simulink model "Modelo_MV_CIGRE_IPSD"  (R2019b)
settings: Solver=FixedStepAuto  StartTime=0.0  StopTime=0.3  FixedStep=Ts  RelTol=1e-3
PreLoadFcn:
  | r_1=0.501
  | l_1=0.716/(60*2*pi)
  | c_1=10e-6/(60*2*pi)
  | r_0=0.817
  | l_0=1.598 /(60*2*pi)
  | c_0=10e-6/(60*2*pi)
  | Sb=50e6
  | Ts=1e-4
InitFcn:
  | r_1=0.501;
  | l_1=0.716/(60*2*pi);
  | c_1=10e-6/(60*2*pi);
  | r_0=0.817;
  | l_0=1.598 /(60*2*pi);
  | c_0=10e-6/(60*2*pi);
  | Sb=50e6;
  | Ts=1e-4;
StartFcn:
  | r_1=0.501
  | l_1=0.716/(60*2*pi)
  | c_1=10e-6/(60*2*pi)
  | r_0=0.817
  | l_0=1.598 /(60*2*pi)
  | c_0=10e-6/(60*2*pi)
  | Sb=50e6
  | Ts=1e-5
undefined symbols (not defined in the file): D1, Delta
libraries: powerlib_meascontrol x112, powerlib x55, simulink x6
(part 1 of 3)
settings Model: Creator=mance  LastModifiedBy=mance

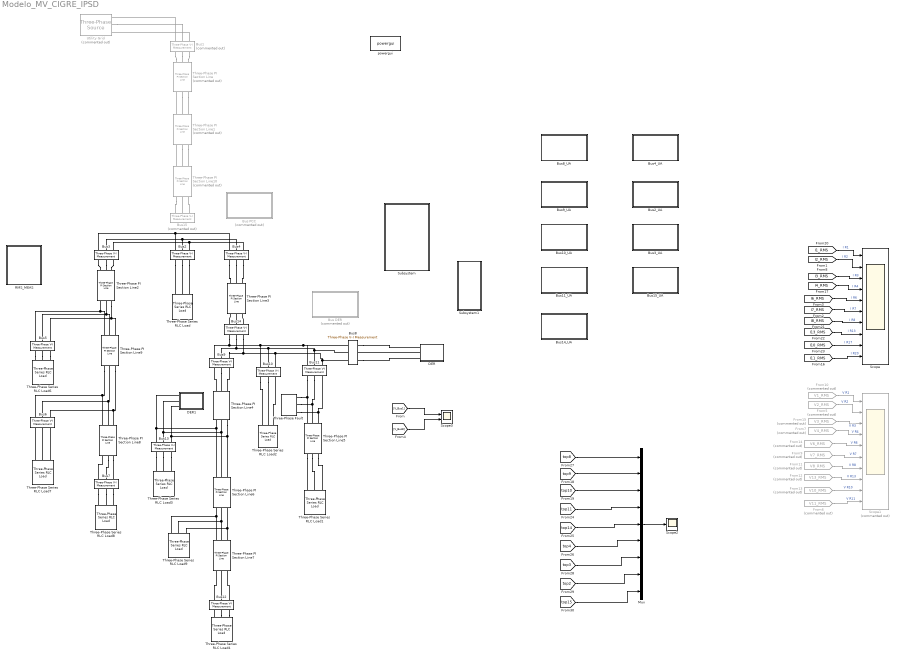
== system Modelo_MV_CIGRE_IPSD ==
  Bus DER : Subsystem  Commented=on
  Bus PCC : Subsystem  Commented=on
  Bus1 : powerlib/Measurements/Three-Phase V-I Measurement  Commented=on  VoltageMeasurement=phase-to-ground  SetLabelV=on  LabelV=V_Bus1  Vpu=on  VpuLL=off  CurrentMeasurement=yes  SetLabelI=on  LabelI=I_Bus1  Ipu=on  Pbase=Sb  Vbase=20e3  OutputType=Complex  PhasorSimulation=off  PSBequivalent=0
      settings: SourceProductName=Simscape Electrical
  Bus10 : powerlib/Measurements/Three-Phase V-I Measurement  VoltageMeasurement=phase-to-ground  SetLabelV=on  LabelV=V_Bus10  Vpu=on  VpuLL=off  CurrentMeasurement=yes  SetLabelI=on  LabelI=I_Bus10  Ipu=on  Pbase=Sb  Vbase=20e3  OutputType=Complex  PhasorSimulation=off  PSBequivalent=0
      settings: SourceProductName=Simscape Electrical
  Bus10_UA : Subsystem
  Bus11 : powerlib/Measurements/Three-Phase V-I Measurement  VoltageMeasurement=phase-to-ground  SetLabelV=on  LabelV=V_Bus11  Vpu=on  VpuLL=off  CurrentMeasurement=yes  SetLabelI=on  LabelI=I_Bus11  Ipu=on  Pbase=Sb  Vbase=20e3  OutputType=Complex  PhasorSimulation=off  PSBequivalent=0
      settings: SourceProductName=Simscape Electrical
  Bus11_UA : Subsystem
  Bus12 : powerlib/Measurements/Three-Phase V-I Measurement  VoltageMeasurement=phase-to-ground  SetLabelV=on  LabelV=V_Bus12  Vpu=on  VpuLL=off  CurrentMeasurement=yes  SetLabelI=on  LabelI=I_Bus12  Ipu=on  Pbase=Sb  Vbase=20e3  OutputType=Complex  PhasorSimulation=off  PSBequivalent=0
      settings: SourceProductName=Simscape Electrical
  Bus13 : powerlib/Measurements/Three-Phase V-I Measurement  VoltageMeasurement=phase-to-ground  SetLabelV=on  LabelV=V_Bus13  Vpu=on  VpuLL=off  CurrentMeasurement=yes  SetLabelI=on  LabelI=I_Bus13  Ipu=on  Pbase=Sb  Vbase=20e3  OutputType=Complex  PhasorSimulation=off  PSBequivalent=0
      settings: SourceProductName=Simscape Electrical
  Bus14 : powerlib/Measurements/Three-Phase V-I Measurement  VoltageMeasurement=phase-to-ground  SetLabelV=on  LabelV=V_Bus14  Vpu=on  VpuLL=off  CurrentMeasurement=yes  SetLabelI=on  LabelI=I_Bus14  Ipu=on  Pbase=Sb  Vbase=20e3  OutputType=Complex  PhasorSimulation=off  PSBequivalent=0
      settings: SourceProductName=Simscape Electrical
  Bus14_UA : Subsystem
  Bus15 : powerlib/Measurements/Three-Phase V-I Measurement  Commented=on  VoltageMeasurement=phase-to-ground  SetLabelV=on  LabelV=V_Bus15  Vpu=on  VpuLL=off  CurrentMeasurement=yes  SetLabelI=on  LabelI=I_Bus15  Ipu=on  Pbase=Sb  Vbase=20e3  OutputType=Complex  PhasorSimulation=off  PSBequivalent=0
      settings: SourceProductName=Simscape Electrical
  Bus15_UA : Subsystem
  Bus2 : powerlib/Measurements/Three-Phase V-I Measurement  VoltageMeasurement=phase-to-ground  SetLabelV=on  LabelV=V_Bus2  Vpu=on  VpuLL=off  CurrentMeasurement=yes  SetLabelI=on  LabelI=I_Bus2  Ipu=on  Pbase=Sb  Vbase=20e3  OutputType=Complex  PhasorSimulation=off  PSBequivalent=0
      settings: SourceProductName=Simscape Electrical
  Bus2_UA : Subsystem
  Bus3 : powerlib/Measurements/Three-Phase V-I Measurement  VoltageMeasurement=phase-to-ground  SetLabelV=on  LabelV=V_Bus3  Vpu=on  VpuLL=off  CurrentMeasurement=yes  SetLabelI=on  LabelI=I_Bus3  Ipu=on  Pbase=Sb  Vbase=20e3  OutputType=Complex  PhasorSimulation=off  PSBequivalent=0
      settings: SourceProductName=Simscape Electrical
  Bus3_UA : Subsystem
  Bus4 : powerlib/Measurements/Three-Phase V-I Measurement  VoltageMeasurement=phase-to-ground  SetLabelV=on  LabelV=V_Bus4  Vpu=on  VpuLL=off  CurrentMeasurement=yes  SetLabelI=on  LabelI=I_Bus4  Ipu=on  Pbase=Sb  Vbase=20e3  OutputType=Complex  PhasorSimulation=off  PSBequivalent=0
      settings: SourceProductName=Simscape Electrical
  Bus4_UA : Subsystem
  Bus5 : powerlib/Measurements/Three-Phase V-I Measurement  VoltageMeasurement=phase-to-ground  SetLabelV=on  LabelV=V_Bus5  Vpu=on  VpuLL=off  CurrentMeasurement=yes  SetLabelI=on  LabelI=I_Bus5  Ipu=on  Pbase=Sb  Vbase=20e3  OutputType=Complex  PhasorSimulation=off  PSBequivalent=0
      settings: SourceProductName=Simscape Electrical
  Bus6 : powerlib/Measurements/Three-Phase V-I Measurement  VoltageMeasurement=phase-to-ground  SetLabelV=on  LabelV=V_Bus6  Vpu=on  VpuLL=off  CurrentMeasurement=yes  SetLabelI=on  LabelI=I_Bus6  Ipu=on  Pbase=Sb  Vbase=20e3  OutputType=Complex  PhasorSimulation=off  PSBequivalent=0
      settings: SourceProductName=Simscape Electrical
  Bus7 : powerlib/Measurements/Three-Phase V-I Measurement  VoltageMeasurement=phase-to-ground  SetLabelV=on  LabelV=V_Bus7  Vpu=on  VpuLL=off  CurrentMeasurement=yes  SetLabelI=on  LabelI=I_Bus7  Ipu=on  Pbase=Sb  Vbase=20e3  OutputType=Complex  PhasorSimulation=off  PSBequivalent=0
      settings: SourceProductName=Simscape Electrical
  Bus8 : powerlib/Measurements/Three-Phase V-I Measurement  VoltageMeasurement=phase-to-ground  SetLabelV=on  LabelV=V_Bus8  Vpu=on  VpuLL=off  CurrentMeasurement=yes  SetLabelI=on  LabelI=I_Bus8  Ipu=on  Pbase=Sb  Vbase=20e3  OutputType=Complex  PhasorSimulation=off  PSBequivalent=0
      settings: SourceProductName=Simscape Electrical
  Bus8_UA : Subsystem
  Bus9 : powerlib/Measurements/Three-Phase V-I Measurement  VoltageMeasurement=phase-to-ground  SetLabelV=on  LabelV=V_Bus9  Vpu=on  VpuLL=off  CurrentMeasurement=yes  SetLabelI=on  LabelI=I_Bus9  Ipu=on  Pbase=Sb  Vbase=20e3  OutputType=Complex  PhasorSimulation=off  PSBequivalent=0
      settings: SourceProductName=Simscape Electrical
  Bus9_UA : Subsystem
  DER : Subsystem
  DER1 : Subsystem
  From10 : From  Commented=on  GotoTag=V1_RMS  TagVisibility=global
  From11 : From  Commented=on  GotoTag=V8_RMS  TagVisibility=global
  From12 : From  Commented=on  GotoTag=V13_RMS  TagVisibility=global
  From13 : From  Commented=on  GotoTag=V10_RMS  TagVisibility=global
  From14 : From  Commented=on  GotoTag=V6_RMS  TagVisibility=global
  From15 : From  Commented=on  GotoTag=V3_RMS  TagVisibility=global
  From5 : From  Commented=on  GotoTag=V2_RMS  TagVisibility=global
  From6 : From  Commented=on  GotoTag=V11_RMS  TagVisibility=global
  From7 : From  Commented=on  GotoTag=V4_RMS  TagVisibility=global
  From9 : From  Commented=on  GotoTag=V7_RMS  TagVisibility=global
  Mux : Mux  Inputs=9
  RMS_MEAS : Subsystem
  Scope : Scope  NumInputPorts=10
  Scope1 : Scope  Commented=on  NumInputPorts=10
  Scope2 : Scope
  Scope3 : Scope  NumInputPorts=2
  Subsystem : Subsystem
  Subsystem1 : Subsystem
  Three-Phase PI Section Line : powerlib/Elements/Three-Phase PI Section Line  Commented=on  LConnTagsString=a|b|c  RConnTagsString=A|B|C  Frequency=60  Resistances=[ r_1 r_0]  Inductances=[ l_1 l_0]  Capacitances=[c_1 c_0]  Length=1.2
      settings: SourceProductName=Simscape Electrical
  Three-Phase PI Section Line1 : powerlib/Elements/Three-Phase PI Section Line  Commented=on  LConnTagsString=a|b|c  RConnTagsString=A|B|C  Frequency=60  Resistances=[r_1 r_0]  Inductances=[l_1 l_0]  Capacitances=[c_1 c_0]  Length=0.5
      settings: SourceProductName=Simscape Electrical
  Three-Phase PI Section Line10 : powerlib/Elements/Three-Phase PI Section Line  Commented=on  LConnTagsString=a|b|c  RConnTagsString=A|B|C  Frequency=60  Resistances=[r_1 r_0]  Inductances=[l_1 l_0]  Capacitances=[c_1 c_0]  Length=0.5
      settings: SourceProductName=Simscape Electrical
  Three-Phase PI Section Line2 : powerlib/Elements/Three-Phase PI Section Line  LConnTagsString=a|b|c  RConnTagsString=A|B|C  Frequency=60  Resistances=[r_1 r_0]  Inductances=[l_1 l_0]  Capacitances=[c_1 c_0]  Length=0.6
      settings: SourceProductName=Simscape Electrical
  Three-Phase PI Section Line3 : powerlib/Elements/Three-Phase PI Section Line  LConnTagsString=a|b|c  RConnTagsString=A|B|C  Frequency=60  Resistances=[r_1 r_0]  Inductances=[l_1 l_0]  Capacitances=[c_1 c_0]  Length=1.3
      settings: SourceProductName=Simscape Electrical
  Three-Phase PI Section Line4 : powerlib/Elements/Three-Phase PI Section Line  LConnTagsString=a|b|c  RConnTagsString=A|B|C  Frequency=60  Resistances=[r_1 r_0]  Inductances=[l_1 l_0]  Capacitances=[c_1 c_0]  Length=0.3
      settings: SourceProductName=Simscape Electrical
  Three-Phase PI Section Line5 : powerlib/Elements/Three-Phase PI Section Line  LConnTagsString=a|b|c  RConnTagsString=A|B|C  Frequency=60  Resistances=[r_1 r_0]  Inductances=[l_1 l_0]  Capacitances=[c_1 c_0]  Length=1.7
      settings: SourceProductName=Simscape Electrical
  Three-Phase PI Section Line6 : powerlib/Elements/Three-Phase PI Section Line  LConnTagsString=a|b|c  RConnTagsString=A|B|C  Frequency=60  Resistances=[r_1 r_0]  Inductances=[l_1 l_0]  Capacitances=[c_1 c_0]  Length=0.8
      settings: SourceProductName=Simscape Electrical
  Three-Phase PI Section Line7 : powerlib/Elements/Three-Phase PI Section Line  LConnTagsString=a|b|c  RConnTagsString=A|B|C  Frequency=60  Resistances=[r_1 r_0]  Inductances=[l_1 l_0]  Capacitances=[c_1 c_0]  Length=0.3
      settings: SourceProductName=Simscape Electrical
  Three-Phase PI Section Line8 : powerlib/Elements/Three-Phase PI Section Line  LConnTagsString=a|b|c  RConnTagsString=A|B|C  Frequency=60  Resistances=[r_1 r_0]  Inductances=[l_1 l_0]  Capacitances=[c_1 c_0]  Length=1.5
      settings: SourceProductName=Simscape Electrical
  Three-Phase PI Section Line9 : powerlib/Elements/Three-Phase PI Section Line  LConnTagsString=a|b|c  RConnTagsString=A|B|C  Frequency=60  Resistances=[r_1 r_0]  Inductances=[l_1 l_0]  Capacitances=[c_1 c_0]  Length=0.6
      settings: SourceProductName=Simscape Electrical
  Three-Phase Series RLC Load : powerlib/Elements/Three-Phase Series RLC Load  LConnTagsString=A|B|C  Configuration=Y (grounded)  NominalVoltage=(20000)  Vabc=[1e3 1e3 1e3]  Vabcp=[1e3 1e3 1e3]  NominalFrequency=60  UnbalancedPower=off  ActivePower=15e3*0.9  InductivePower=sqrt(15e3^2-(15e3*0.9)^2)  CapacitivePower=0  Pabc=[10e3 9e3 11e3]  QLabc=[100 90 110]  QCabc=[100 90 110]  Pabcp=[10e3 9e3 11e3]  QLabcp=[100 90 110]  QCabcp=[100 90 110]  Measurements=None  LoadType=constant PQ
      settings: SourceProductName=Simscape Electrical
  Three-Phase Series RLC Load1 : powerlib/Elements/Three-Phase Series RLC Load  LConnTagsString=A|B|C  Configuration=Y (grounded)  NominalVoltage=(20000)  Vabc=[1e3 1e3 1e3]  Vabcp=[1e3 1e3 1e3]  NominalFrequency=60  UnbalancedPower=off  ActivePower=50e3*0.95*0.7  InductivePower=sqrt(50e3^2-(50e3*0.95)^2)*0.7  CapacitivePower=0  Pabc=[10e3 9e3 11e3]  QLabc=[100 90 110]  QCabc=[100 90 110]  Pabcp=[10e3 9e3 11e3]  QLabcp=[100 90 110]  QCabcp=[100 90 110]  Measurements=None  LoadType=constant PQ
      settings: SourceProductName=Simscape Electrical
  Three-Phase Series RLC Load2 : powerlib/Elements/Three-Phase Series RLC Load  LConnTagsString=A|B|C  Configuration=Y (grounded)  NominalVoltage=(20000)  Vabc=[1e3 1e3 1e3]  Vabcp=[1e3 1e3 1e3]  NominalFrequency=60  UnbalancedPower=off  ActivePower=10e3*0.95*0.7  InductivePower=sqrt(10e3^2-(10e3*0.95)^2)*0.7  CapacitivePower=0  Pabc=[10e3 9e3 11e3]  QLabc=[100 90 110]  QCabc=[100 90 110]  Pabcp=[10e3 9e3 11e3]  QLabcp=[100 90 110]  QCabcp=[100 90 110]  Measurements=None  LoadType=constant PQ
      settings: SourceProductName=Simscape Electrical
  Three-Phase Series RLC Load3 : powerlib/Elements/Three-Phase Series RLC Load  LConnTagsString=A|B|C  Configuration=Y (grounded)  NominalVoltage=(20000)  Vabc=[1e3 1e3 1e3]  Vabcp=[1e3 1e3 1e3]  NominalFrequency=60  UnbalancedPower=off  ActivePower=50e3*0.95*0.7  InductivePower=sqrt(50e3^2-(50e3*0.95)^2)*0.7  CapacitivePower=0  Pabc=[10e3 9e3 11e3]  QLabc=[100 90 110]  QCabc=[100 90 110]  Pabcp=[10e3 9e3 11e3]  QLabcp=[100 90 110]  QCabcp=[100 90 110]  Measurements=None  LoadType=constant PQ
      settings: SourceProductName=Simscape Electrical
  Three-Phase Series RLC Load4 : powerlib/Elements/Three-Phase Series RLC Load  LConnTagsString=A|B|C  Configuration=Y (grounded)  NominalVoltage=(20000)  Vabc=[1e3 1e3 1e3]  Vabcp=[1e3 1e3 1e3]  NominalFrequency=60  UnbalancedPower=off  ActivePower=10e3*0.95*0.7  InductivePower=sqrt(10e3^2-(10e3*0.95)^2)*0.7  CapacitivePower=0  Pabc=[10e3 9e3 11e3]  QLabc=[100 90 110]  QCabc=[100 90 110]  Pabcp=[10e3 9e3 11e3]  QLabcp=[100 90 110]  QCabcp=[100 90 110]  Measurements=None  LoadType=constant PQ
      settings: SourceProductName=Simscape Electrical
  Three-Phase Series RLC Load6 : powerlib/Elements/Three-Phase Series RLC Load  LConnTagsString=A|B|C  Configuration=Y (grounded)  NominalVoltage=(20000)  Vabc=[1e3 1e3 1e3]  Vabcp=[1e3 1e3 1e3]  NominalFrequency=60  UnbalancedPower=off  ActivePower=15e3*0.9  InductivePower=sqrt(15e3^2-(15e3*0.9)^2)  CapacitivePower=0  Pabc=[10e3 9e3 11e3]  QLabc=[100 90 110]  QCabc=[100 90 110]  Pabcp=[10e3 9e3 11e3]  QLabcp=[100 90 110]  QCabcp=[100 90 110]  Measurements=None  LoadType=constant PQ
      settings: SourceProductName=Simscape Electrical
  Three-Phase Series RLC Load7 : powerlib/Elements/Three-Phase Series RLC Load  LConnTagsString=A|B|C  Configuration=Y (grounded)  NominalVoltage=(20000)  Vabc=[1e3 1e3 1e3]  Vabcp=[1e3 1e3 1e3]  NominalFrequency=60  UnbalancedPower=off  ActivePower=10e3*0.95  InductivePower=sqrt(10e3^2-(10e3*0.95)^2)  CapacitivePower=0  Pabc=[10e3 9e3 11e3]  QLabc=[100 90 110]  QCabc=[100 90 110]  Pabcp=[10e3 9e3 11e3]  QLabcp=[100 90 110]  QCabcp=[100 90 110]  Measurements=None  LoadType=constant PQ
      settings: SourceProductName=Simscape Electrical
  Three-Phase Series RLC Load8 : powerlib/Elements/Three-Phase Series RLC Load  LConnTagsString=A|B|C  Configuration=Y (grounded)  NominalVoltage=(20000)  Vabc=[1e3 1e3 1e3]  Vabcp=[1e3 1e3 1e3]  NominalFrequency=60  UnbalancedPower=off  ActivePower=50e3*0.95  InductivePower=sqrt(50e3^2-(50e3*0.95)^2)  CapacitivePower=0  Pabc=[10e3 9e3 11e3]  QLabc=[100 90 110]  QCabc=[100 90 110]  Pabcp=[10e3 9e3 11e3]  QLabcp=[100 90 110]  QCabcp=[100 90 110]  Measurements=None  LoadType=constant PQ
      settings: SourceProductName=Simscape Electrical
  Three-Phase Series RLC Load9 : powerlib/Elements/Three-Phase Series RLC Load  LConnTagsString=A|B|C  Configuration=Y (grounded)  NominalVoltage=(20000)  Vabc=[1e3 1e3 1e3]  Vabcp=[1e3 1e3 1e3]  NominalFrequency=60  UnbalancedPower=off  ActivePower=15e3*0.9  InductivePower=sqrt(15e3^2-(15e3*0.9)^2)*0.7  CapacitivePower=0  Pabc=[10e3 9e3 11e3]  QLabc=[100 90 110]  QCabc=[100 90 110]  Pabcp=[10e3 9e3 11e3]  QLabcp=[100 90 110]  QCabcp=[100 90 110]  Measurements=None  LoadType=constant PQ
      settings: SourceProductName=Simscape Electrical
  Three-Phase Fault : powerlib/Elements/Three-Phase Fault  InitialStates=0  FaultA=on  FaultB=on  FaultC=on  GroundFault=on  SwitchTimes=0.11  External=off  SwitchStatus=NaN  FaultResistance=1  GroundResistance=0.01  SnubberResistance=1e6  SnubberCapacitance=inf  Measurements=None
      settings: SourceProductName=Simscape Electrical
  Utility Grid : powerlib/Electrical Sources/Three-Phase Source  Commented=on  InternalConnection=Yg  VoltagePhases=off  Voltage=20e3  PhaseAngle=0  Voltage_phases=[89.8e3 89.8e3 89.8e3]/sqrt(2)  PhaseAngles_phases=[0 -120 +120]  Frequency=60  NonIdealSource=on  SpecifyImpedance=on  Resistance=0.01  Inductance=1.58e-3  ShortCircuitLevel=60e6  BaseVoltage=20e3  XRratio=7  BusType=swing  Pref=10e3  Qref=0  Prefabc=[10e3, 10e3, 10e3]  Qrefabc=[0, 0, 0]  Qmin=-inf  Qmax=inf
      settings: SourceProductName=Simscape Electrical
  powergui : powerlib/powergui  Priority=1  SimulationMode=Discrete  SampleTime=Ts  frequency=60  Iterations=50  frequencyindice=60  Pbase=100e6  ErrMax=0.0001  UnitsV=kV  UnitsW=MW  buscounter=0  FunctionMessages=off  echomessages=off  EnableUseOfTLC=off  CurrentSourceSwitches=off  DisableSnubberDevices=off  DisableRonSwitches=off  DisableVfSwitches=off  DisplayEquations=off  AutomaticDiscreteSolvers=off  SolverType=Tustin/Backward Euler (TBE)  Interpol=off  ExternalGateDelay=off  methode=off  Ts=100  x0status=blocks  SPID=on  SwTol=0  HookPort=off  NonlinearTolerance=1e-4  nMaxIteration=100  ContinueOnMaxIteration=off  RestoreLinks=warning  ResistiveCurrentMeasurement=off  Frange=[0:2:500]  Ylog=off  Xlog=on  ShowGrid=off  save=off  variable=ZData  structure=0  ZoomFFT=off  StartTime=0.0  cycles=1  DisplayStyle=1  fundamental=60  FreqAxis=off  MaxFrequency=1000  frequencyindicesteady=1  RmsSteady=1  display=off
      settings: SourceProductName=Simscape Electrical
  wires:
  [I2_RMS] -> Scope/2  "I R2"
  [I11_RMS] -> Scope/10  "I R20"
  [I1_RMS] -> Scope/1  "I R1"
  [I3_RMS] -> Scope/3  "I R3"
  [I4_RMS] -> Scope/4  "I R4"
  [I6_RMS] -> Scope/5  "I R6"
  [I7_RMS] -> Scope/6  "I R7"
  [I8_RMS] -> Scope/7  "I R8"
  [I13_RMS] -> Scope/8  "I R13"
  [I10_RMS] -> Scope/9  "I R17"
  [V_Bus8] -> Scope3/2
  [V_Bus1] -> Scope3/1
  From13/1 -> Scope1/9  "V R10"
  From12/1 -> Scope1/8  "V R13"
  From11/1 -> Scope1/7  "V R8"
  From9/1 -> Scope1/6  "V R7"
  From14/1 -> Scope1/5  "V R6"
  From7/1 -> Scope1/4  "V R4"
  From15/1 -> Scope1/3  "V R3"
  From10/1 -> Scope1/1  "V R1"
  From6/1 -> Scope1/10  "V R11"
  From5/1 -> Scope1/2  "V R2"
  [top8] -> Mux/1
  [top9] -> Mux/2
  [top10] -> Mux/3
  [top11] -> Mux/4
  [top14] -> Mux/5
  [top4] -> Mux/6
  [top3] -> Mux/7
  [top2] -> Mux/8
  [top15] -> Mux/9
  Mux/1 -> Scope2/1
  connections:
  Three-Phase PI Section Line1/LConn1 -- Three-Phase PI Section Line/RConn1
  Three-Phase PI Section Line/RConn3 -- Three-Phase PI Section Line1/LConn3
  Three-Phase PI Section Line5/RConn1 -- Three-Phase Series RLC Load1/LConn1
  Three-Phase PI Section Line5/RConn3 -- Three-Phase Series RLC Load1/LConn3
  Three-Phase PI Section Line/RConn2 -- Three-Phase PI Section Line1/LConn2
  Bus8/LConn2 -- Bus11/LConn2 -- Bus14/LConn2 -- Bus9/LConn2 -- Bus10/LConn2
  Bus8/LConn1 -- Bus11/LConn1 -- Bus9/LConn1 -- Bus14/LConn1 -- Bus10/LConn1
  Bus8/LConn3 -- Bus11/LConn3 -- Bus14/LConn3 -- Bus9/LConn3 -- Bus10/LConn3
  Three-Phase PI Section Line5/RConn2 -- Three-Phase Series RLC Load1/LConn2
  Three-Phase PI Section Line6/LConn2 -- DER1/LConn2 -- Bus13/LConn2 -- Three-Phase PI Section Line4/RConn2
  Three-Phase PI Section Line6/LConn1 -- Three-Phase PI Section Line4/RConn1 -- DER1/LConn1 -- Bus13/LConn1
  Three-Phase PI Section Line4/RConn3 -- DER1/LConn3 -- Bus13/LConn3 -- Three-Phase PI Section Line6/LConn3
  Three-Phase PI Section Line6/RConn1 -- Three-Phase Series RLC Load9/LConn1 -- Three-Phase PI Section Line7/LConn1
  Three-Phase PI Section Line6/RConn2 -- Three-Phase Series RLC Load9/LConn2 -- Three-Phase PI Section Line7/LConn2
  Three-Phase PI Section Line6/RConn3 -- Three-Phase Series RLC Load9/LConn3 -- Three-Phase PI Section Line7/LConn3
  Bus12/LConn2 -- Three-Phase PI Section Line7/RConn2
  Bus12/LConn1 -- Three-Phase PI Section Line7/RConn1
  Bus12/LConn3 -- Three-Phase PI Section Line7/RConn3
  Bus12/RConn2 -- Three-Phase Series RLC Load4/LConn2
  Three-Phase Series RLC Load4/LConn1 -- Bus12/RConn1
  Bus12/RConn3 -- Three-Phase Series RLC Load4/LConn3
  Bus5/LConn1 -- Three-Phase PI Section Line9/LConn1 -- Three-Phase PI Section Line2/RConn1
  Three-Phase PI Section Line2/RConn3 -- Three-Phase PI Section Line9/LConn3 -- Bus5/LConn3
  Bus5/LConn2 -- Three-Phase PI Section Line9/LConn2 -- Three-Phase PI Section Line2/RConn2
  Bus7/LConn1 -- Three-Phase PI Section Line8/RConn1
  Bus7/RConn2 -- Three-Phase Series RLC Load8/LConn2
  Bus7/RConn1 -- Three-Phase Series RLC Load8/LConn1
  Bus7/RConn3 -- Three-Phase Series RLC Load8/LConn3
  Bus1/LConn1 -- Utility Grid/RConn1
  Bus1/LConn3 -- Utility Grid/RConn3
  Three-Phase PI Section Line10/LConn1 -- Three-Phase PI Section Line1/RConn1
  Three-Phase PI Section Line1/RConn2 -- Three-Phase PI Section Line10/LConn2
  Three-Phase PI Section Line1/RConn3 -- Three-Phase PI Section Line10/LConn3
  Utility Grid/RConn2 -- Bus1/LConn2
  Bus1/RConn1 -- Three-Phase PI Section Line/LConn1
  Bus1/RConn2 -- Three-Phase PI Section Line/LConn2
  Bus1/RConn3 -- Three-Phase PI Section Line/LConn3
  Bus4/LConn1 -- Bus2/LConn1 -- Bus3/LConn1
  Bus4/LConn2 -- Bus3/LConn2 -- Bus2/LConn2
  Bus4/LConn3 -- Bus3/LConn3 -- Bus2/LConn3
  Bus2/RConn1 -- Three-Phase Series RLC Load/LConn1
  Bus2/RConn2 -- Three-Phase Series RLC Load/LConn2
  Bus2/RConn3 -- Three-Phase Series RLC Load/LConn3
  Bus3/RConn1 -- Three-Phase PI Section Line2/LConn1
  Bus3/RConn2 -- Three-Phase PI Section Line2/LConn2
  Bus3/RConn3 -- Three-Phase PI Section Line2/LConn3
  Bus4/RConn1 -- Three-Phase PI Section Line3/LConn1
  Bus4/RConn2 -- Three-Phase PI Section Line3/LConn2
  Bus4/RConn3 -- Three-Phase PI Section Line3/LConn3
  Bus5/RConn1 -- Three-Phase Series RLC Load6/LConn1
  Bus5/RConn2 -- Three-Phase Series RLC Load6/LConn2
  Bus5/RConn3 -- Three-Phase Series RLC Load6/LConn3
  Three-Phase PI Section Line9/RConn3 -- Bus6/LConn3 -- Three-Phase PI Section Line8/LConn3
  Three-Phase PI Section Line8/LConn2 -- Bus6/LConn2 -- Three-Phase PI Section Line9/RConn2
  Three-Phase PI Section Line9/RConn1 -- Three-Phase PI Section Line8/LConn1 -- Bus6/LConn1
  Three-Phase Series RLC Load7/LConn1 -- Bus6/RConn1
  Three-Phase Series RLC Load7/LConn2 -- Bus6/RConn2
  Three-Phase Series RLC Load7/LConn3 -- Bus6/RConn3
  Three-Phase PI Section Line8/RConn2 -- Bus7/LConn2
  Three-Phase PI Section Line8/RConn3 -- Bus7/LConn3
  Bus10/RConn2 -- Three-Phase Series RLC Load2/LConn2
  Three-Phase Series RLC Load2/LConn3 -- Bus10/RConn3
  Bus10/RConn1 -- Three-Phase Series RLC Load2/LConn1
  Bus13/RConn2 -- Three-Phase Series RLC Load3/LConn2
  Bus13/RConn1 -- Three-Phase Series RLC Load3/LConn1
  Bus13/RConn3 -- Three-Phase Series RLC Load3/LConn3
  Bus11/RConn2 -- Three-Phase PI Section Line5/LConn2 -- Three-Phase Fault/LConn2
  Bus11/RConn1 -- Three-Phase Fault/LConn1 -- Three-Phase PI Section Line5/LConn1
  Three-Phase PI Section Line5/LConn3 -- Three-Phase Fault/LConn3 -- Bus11/RConn3
  Bus9/RConn2 -- Three-Phase PI Section Line4/LConn2
  Three-Phase PI Section Line4/LConn1 -- Bus9/RConn1
  Three-Phase PI Section Line4/LConn3 -- Bus9/RConn3
  Bus8/RConn1 -- DER/LConn1
  DER/LConn2 -- Bus8/RConn2
  Bus8/RConn3 -- DER/LConn3
  Bus14/RConn1 -- Three-Phase PI Section Line3/RConn1
  Bus14/RConn2 -- Three-Phase PI Section Line3/RConn2
  Bus14/RConn3 -- Three-Phase PI Section Line3/RConn3
  Bus15/RConn3 -- Three-Phase PI Section Line10/RConn3
  Bus15/RConn2 -- Three-Phase PI Section Line10/RConn2
  Three-Phase PI Section Line10/RConn1 -- Bus15/RConn1

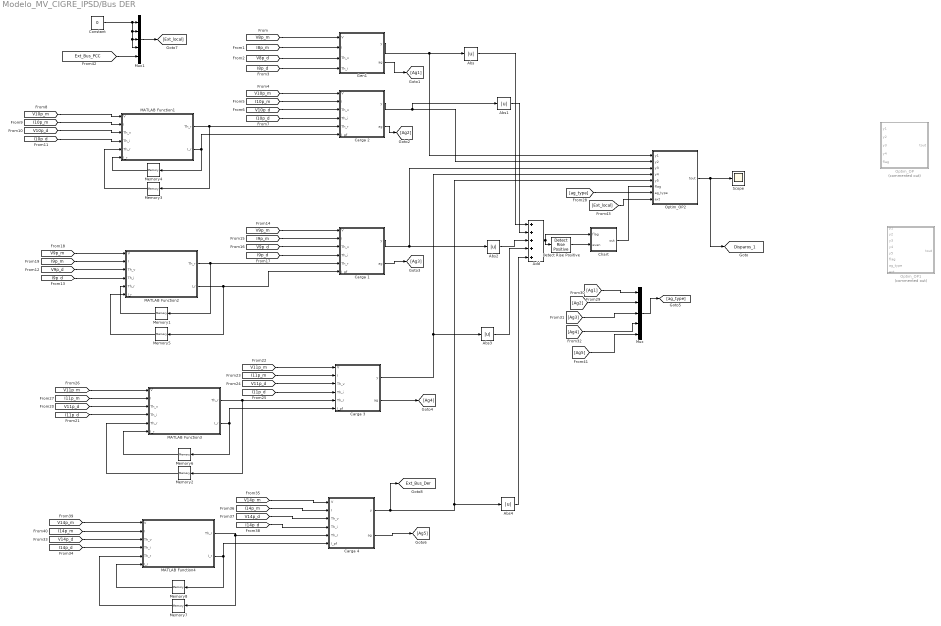
== system Modelo_MV_CIGRE_IPSD/Bus DER ==
  Abs{,1..4} (5 alike) : Abs
  Add : Sum  Inputs=+++++
  Carga 1 : MATLAB Function  TreatAsAtomicUnit=on
  Carga 2 : MATLAB Function  TreatAsAtomicUnit=on
  Carga 3 : MATLAB Function  TreatAsAtomicUnit=on
  Carga 4 : MATLAB Function  TreatAsAtomicUnit=on
  Chart : Stateflow chart  BlockKeywords=__PRM__SERIALIZED__DATA__:Stateflow Chart,Stateflow Diagram  TreatAsAtomicUnit=on
  Constant : Constant  Value=0
  Detect Rise Positive : simulink/Logic and Bit Operations/Detect Rise Positive  vinit=0  OutDataTypeStr=boolean
  Gen1 : MATLAB Function  TreatAsAtomicUnit=on
  MATLAB Function1 : MATLAB Function  TreatAsAtomicUnit=on
  MATLAB Function2 : MATLAB Function  TreatAsAtomicUnit=on
  MATLAB Function3 : MATLAB Function  TreatAsAtomicUnit=on
  MATLAB Function4 : MATLAB Function  TreatAsAtomicUnit=on
  Memory{1..8} (8 alike) : Memory
  Mux : Mux  Inputs=5
  Mux1 : Mux  Inputs=5
  Optim_OP : MATLAB Function  Commented=on  TreatAsAtomicUnit=on
  Optim_OP1 : MATLAB Function  Commented=on  TreatAsAtomicUnit=on
  Optim_OP2 : MATLAB Function  TreatAsAtomicUnit=on
  Scope : Scope
  tag scope: Disparos_1=global, Ext_Bus_Der=global
  wires:
  [V8p_m] -> Gen1/1(V)
  [I8p_m] -> Gen1/2(I)
  [V8p_d] -> Gen1/3(Th_v)
  [I8p_d] -> Gen1/4(Th_i)
  [V10p_m] -> Carga 2/1(V)
  [I10p_m] -> Carga 2/2(I)
  [V10p_d] -> Carga 2/3(Th_v)
  [I10p_d] -> Carga 2/4(Th_i)
  [I10p_d] -> MATLAB Function1/4(Th_i)
  [V10p_d] -> MATLAB Function1/3(Th_v)
  [I10p_m] -> MATLAB Function1/2(I)
  [V10p_m] -> MATLAB Function1/1(V)
  [I9p_d] -> Carga 1/4(Th_i)
  [V9p_d] -> Carga 1/3(Th_v)
  [I9p_m] -> Carga 1/2(I)
  [V9p_m] -> Carga 1/1(V)
  Memory2/1 -> MATLAB Function3/5("Th_r ")
  [V11p_m] -> Carga 3/1(V)
  [I11p_m] -> Carga 3/2(I)
  [V11p_d] -> Carga 3/3(Th_v)
  [I11p_d] -> Carga 3/4(Th_i)
  [I11p_d] -> MATLAB Function3/4(Th_i)
  [V11p_d] -> MATLAB Function3/3(Th_v)
  [I11p_m] -> MATLAB Function3/2(I)
  [V11p_m] -> MATLAB Function3/1(V)
  Carga 2/1(y) -> Optim_OP2/2(y2), Abs1/1
  Carga 1/1(y) -> Optim_OP2/3(y3), Abs2/1
  Carga 3/1(y) -> Optim_OP2/4(y4), Abs3/1
  Gen1/1(y) -> Optim_OP2/1(y1), Abs/1
  Optim_OP2/1(tout) -> [Disparos_1], Scope/1
  Abs/1 -> Add/1
  Abs1/1 -> Add/2
  Abs2/1 -> Add/3
  Abs3/1 -> Add/4
  Add/1 -> Chart/1(flag), Detect Rise Positive/1
  Chart/1(out) -> Optim_OP2/6(flag)
  Detect Rise Positive/1 -> Chart/2(even)
  Gen1/2(ag) -> [Ag1]
  Carga 2/2(ag) -> [Ag2]
  Carga 1/2(ag) -> [Ag3]
  Carga 3/2(ag) -> [Ag4]
  Mux/1 -> [ag_type]
  [ag_type] -> Optim_OP2/7(ag_type)
  [Ag1] -> Mux/1
  [Ag2] -> Mux/2
  [Ag3] -> Mux/3
  [Ag4] -> Mux/4
  Memory4/1 -> MATLAB Function1/6("I_r ")
  MATLAB Function1/2(I_r) -> Memory4/1, Carga 2/6(I_pf)
  MATLAB Function1/1(Th_r) -> Memory3/1, Carga 2/5(Th_r)
  Memory3/1 -> MATLAB Function1/5("Th_r ")
  [V9p_m] -> MATLAB Function2/1(V)
  [I9p_m] -> MATLAB Function2/2(I)
  [V9p_d] -> MATLAB Function2/3(Th_v)
  [I9p_d] -> MATLAB Function2/4(Th_i)
  MATLAB Function2/1(Th_r) -> Memory1/1, Carga 1/5(Th_r)
  MATLAB Function2/2(I_r) -> Memory5/1, Carga 1/6(I_pf)
  Memory1/1 -> MATLAB Function2/5("Th_r ")
  Memory5/1 -> MATLAB Function2/6("I_r ")
  MATLAB Function3/1(Th_r) -> Memory2/1, Carga 3/5(Th_r)
  Memory6/1 -> MATLAB Function3/6("I_r ")
  MATLAB Function3/2(I_r) -> Carga 3/6(I_pf), Memory6/1
  MATLAB Function4/2(I_r) -> Memory8/1, Carga 4/6(I_pf)
  Memory8/1 -> MATLAB Function4/6("I_r ")
  MATLAB Function4/1(Th_r) -> Carga 4/5(Th_r), Memory7/1
  Carga 4/2(ag) -> [Ag5]
  [V14p_m] -> MATLAB Function4/1(V)
  [I14p_m] -> MATLAB Function4/2(I)
  [V14p_d] -> MATLAB Function4/3(Th_v)
  [I14p_d] -> MATLAB Function4/4(Th_i)
  [I14p_d] -> Carga 4/4(Th_i)
  [V14p_d] -> Carga 4/3(Th_v)
  [I14p_m] -> Carga 4/2(I)
  [V14p_m] -> Carga 4/1(V)
  Memory7/1 -> MATLAB Function4/5("Th_r ")
  Abs4/1 -> Add/5
  Carga 4/1(y) -> [Ext_Bus_Der], Optim_OP2/5(y5), Abs4/1
  [Ag5] -> Mux/5
  Constant/1 -> Mux1/4, Mux1/3, Mux1/2, Mux1/1
  [Ext_Bus_PCC] -> Mux1/5
  Mux1/1 -> [Ext_local]
  [Ext_local] -> Optim_OP2/8(ext)

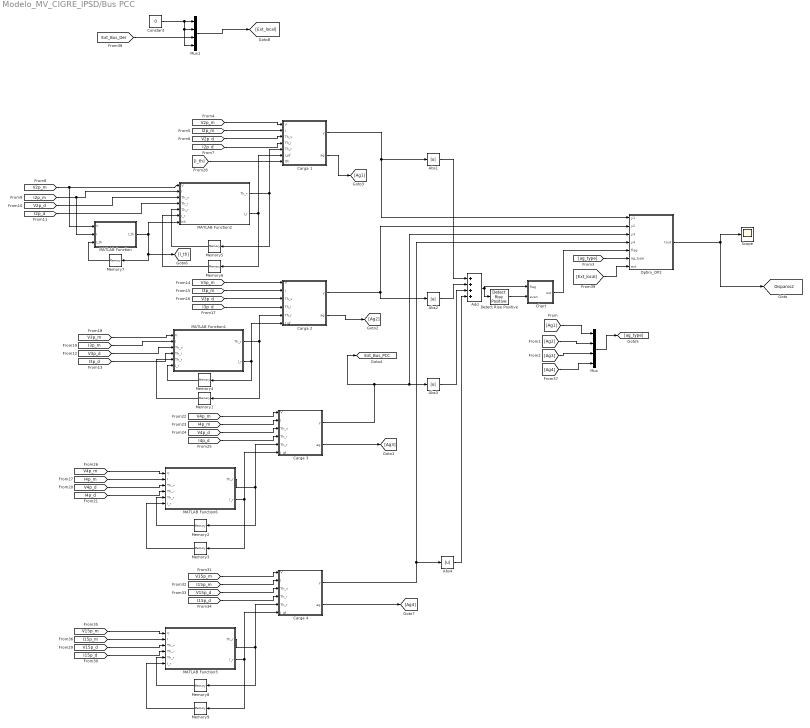
== system Modelo_MV_CIGRE_IPSD/Bus PCC ==
  Abs{1..4} (4 alike) : Abs
  Add : Sum  Inputs=++++
  Carga 1 : MATLAB Function  TreatAsAtomicUnit=on
  Carga 2 : MATLAB Function  TreatAsAtomicUnit=on
  Carga 3 : MATLAB Function  TreatAsAtomicUnit=on
  Carga 4 : MATLAB Function  TreatAsAtomicUnit=on
  Chart : Stateflow chart  BlockKeywords=__PRM__SERIALIZED__DATA__:Stateflow Chart,Stateflow Diagram  TreatAsAtomicUnit=on
  Constant : Constant  Value=0
  Detect Rise Positive : simulink/Logic and Bit Operations/Detect Rise Positive  vinit=0  OutDataTypeStr=boolean
  MATLAB Function : MATLAB Function  TreatAsAtomicUnit=on
  MATLAB Function1 : MATLAB Function  TreatAsAtomicUnit=on
  MATLAB Function2 : MATLAB Function  TreatAsAtomicUnit=on
  MATLAB Function3 : MATLAB Function  TreatAsAtomicUnit=on
  MATLAB Function6 : MATLAB Function  TreatAsAtomicUnit=on
  Memory{1..9} (9 alike) : Memory
  Mux : Mux
  Mux1 : Mux
  Optim_OP2 : MATLAB Function  TreatAsAtomicUnit=on
  Scope : Scope
  tag scope: Disparos2=global, Ext_Bus_PCC=global
  wires:
  Detect Rise Positive/1 -> Chart/2(even)
  Add/1 -> Chart/1(flag), Detect Rise Positive/1
  Optim_OP2/1(tout) -> Scope/1, [Disparos2]
  Carga 3/1(y) -> [Ext_Bus_PCC], Optim_OP2/3(y3), Abs3/1
  Carga 2/1(y) -> Optim_OP2/2(y2), Abs2/1
  Carga 1/1(y) -> Optim_OP2/1(y1), Abs1/1
  [V4p_m] -> MATLAB Function6/1(V)
  [I4p_m] -> MATLAB Function6/2(I)
  [V4p_d] -> MATLAB Function6/3(Th_v)
  [I4p_d] -> MATLAB Function6/4(Th_i)
  [I4p_d] -> Carga 3/4(Th_i)
  [V4p_d] -> Carga 3/3(Th_v)
  [I4p_m] -> Carga 3/2(I)
  [V4p_m] -> Carga 3/1(V)
  Memory2/1 -> MATLAB Function6/5("Th_r ")
  MATLAB Function6/1(Th_r) -> Carga 3/5(Th_r), Memory2/1
  MATLAB Function1/1(Th_r) -> Carga 2/5(Th_r), Memory1/1
  Memory1/1 -> MATLAB Function1/5("Th_r ")
  [V3p_m] -> Carga 2/1(V)
  [I3p_m] -> Carga 2/2(I)
  [V3p_d] -> Carga 2/3(Th_v)
  [I3p_d] -> Carga 2/4(Th_i)
  [I3p_d] -> MATLAB Function1/4(Th_i)
  [I3p_m] -> MATLAB Function1/2(I)
  [V3p_m] -> MATLAB Function1/1(V)
  [V2p_m] -> MATLAB Function/1(V), MATLAB Function2/1(V)
  [I2p_m] -> MATLAB Function/2(I), MATLAB Function2/2(I)
  [V2p_d] -> MATLAB Function2/3(Th_v)
  [I2p_d] -> MATLAB Function2/4(Th_i)
  [I2p_d] -> Carga 1/4(Th_i)
  [V2p_d] -> Carga 1/3(Th_v)
  [I2p_m] -> Carga 1/2(I)
  [V2p_m] -> Carga 1/1(V)
  Abs1/1 -> Add/1
  Abs2/1 -> Add/2
  Abs3/1 -> Add/3
  Carga 3/2(ag) -> [Ag3]
  Carga 2/2(ag) -> [Ag2]
  Carga 1/2(ag) -> [Ag1]
  [Ag2] -> Mux/2
  [Ag3] -> Mux/3
  [Ag1] -> Mux/1
  Mux/1 -> [ag_type]
  [ag_type] -> Optim_OP2/6(ag_type)
  MATLAB Function6/2(I_r) -> Carga 3/6(I_pf), Memory3/1
  Memory3/1 -> MATLAB Function6/6("I_r ")
  [V3p_d] -> MATLAB Function1/3(Th_v)
  Memory4/1 -> MATLAB Function1/6("I_r ")
  MATLAB Function1/2(I_r) -> Carga 2/6(I_pf), Memory4/1
  Memory6/1 -> MATLAB Function2/6("I_r ")
  Memory5/1 -> MATLAB Function2/5("Th_r ")
  MATLAB Function2/1(Th_r) -> Carga 1/5(Th_r), Memory5/1
  MATLAB Function2/2(I_r) -> Carga 1/6(I_pf), Memory6/1
  MATLAB Function/1(I_th) -> [I_th], Memory7/1, MATLAB Function2/7(Ith)
  Memory7/1 -> MATLAB Function/3("I_th ")
  [I_th] -> Carga 1/7(Ith)
  Chart/1(out) -> Optim_OP2/5(flag)
  Memory9/1 -> MATLAB Function3/6("I_r ")
  MATLAB Function3/2(I_r) -> Memory9/1, Carga 4/6(I_pf)
  Carga 4/2(ag) -> [Ag4]
  MATLAB Function3/1(Th_r) -> Memory8/1, Carga 4/5(Th_r)
  Memory8/1 -> MATLAB Function3/5("Th_r ")
  [V15p_m] -> Carga 4/1(V)
  [I15p_m] -> Carga 4/2(I)
  [V15p_d] -> Carga 4/3(Th_v)
  [I15p_d] -> Carga 4/4(Th_i)
  [I15p_d] -> MATLAB Function3/4(Th_i)
  [V15p_d] -> MATLAB Function3/3(Th_v)
  [I15p_m] -> MATLAB Function3/2(I)
  [V15p_m] -> MATLAB Function3/1(V)
  [Ag4] -> Mux/4
  Abs4/1 -> Add/4
  Carga 4/1(y) -> Optim_OP2/4(y4), Abs4/1
  [Ext_Bus_Der] -> Mux1/3
  Constant/1 -> Mux1/4, Mux1/2, Mux1/1
  Mux1/1 -> [Ext_local]
  [Ext_local] -> Optim_OP2/7(ext)

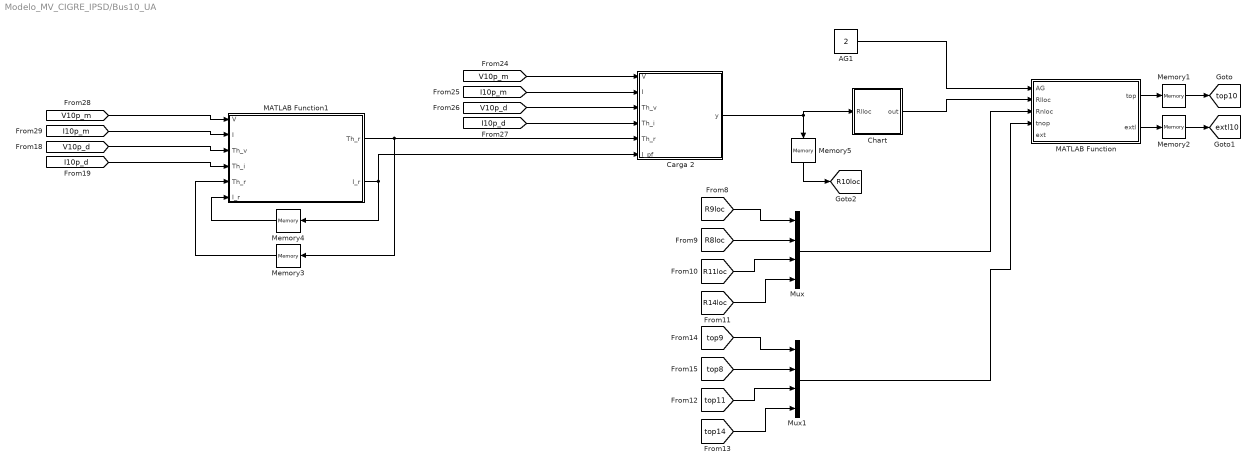
== system Modelo_MV_CIGRE_IPSD/Bus10_UA ==
  AG1 : Constant  Value=2
  Carga 2 : MATLAB Function  TreatAsAtomicUnit=on
  Chart : Stateflow chart  BlockKeywords=__PRM__SERIALIZED__DATA__:Stateflow Chart,Stateflow Diagram  TreatAsAtomicUnit=on
  MATLAB Function : MATLAB Function  TreatAsAtomicUnit=on
  MATLAB Function1 : MATLAB Function  TreatAsAtomicUnit=on
  Memory{1..5} (5 alike) : Memory
  Mux : Mux
  Mux1 : Mux
  tag scope: R10loc=global, extl10=global, top10=global
  wires:
  AG1/1 -> MATLAB Function/1(AG)
  MATLAB Function/1(top) -> Memory1/1
  MATLAB Function/2(extl) -> Memory2/1
  MATLAB Function1/2(I_r) -> Carga 2/6(I_pf), Memory4/1
  Memory3/1 -> MATLAB Function1/5("Th_r ")
  [V10p_d] -> MATLAB Function1/3(Th_v)
  [I10p_d] -> Carga 2/4(Th_i)
  Memory4/1 -> MATLAB Function1/6("I_r ")
  [I10p_d] -> MATLAB Function1/4(Th_i)
  [V10p_d] -> Carga 2/3(Th_v)
  MATLAB Function1/1(Th_r) -> Carga 2/5(Th_r), Memory3/1
  [I10p_m] -> MATLAB Function1/2(I)
  [V10p_m] -> Carga 2/1(V)
  [I10p_m] -> Carga 2/2(I)
  [V10p_m] -> MATLAB Function1/1(V)
  Carga 2/1(y) -> Chart/1(Rlloc), Memory5/1
  [top9] -> Mux1/1
  [top8] -> Mux1/2
  [top11] -> Mux1/3
  Mux/1 -> MATLAB Function/3(Rnloc)
  [top14] -> Mux1/4
  [R8loc] -> Mux/2
  [R11loc] -> Mux/3
  [R9loc] -> Mux/1
  Mux1/1 -> MATLAB Function/4(tnop)
  [R14loc] -> Mux/4
  Memory1/1 -> [top10]
  Memory2/1 -> [extl10]
  Memory5/1 -> [R10loc]
  Chart/1(out) -> MATLAB Function/2(Rlloc)

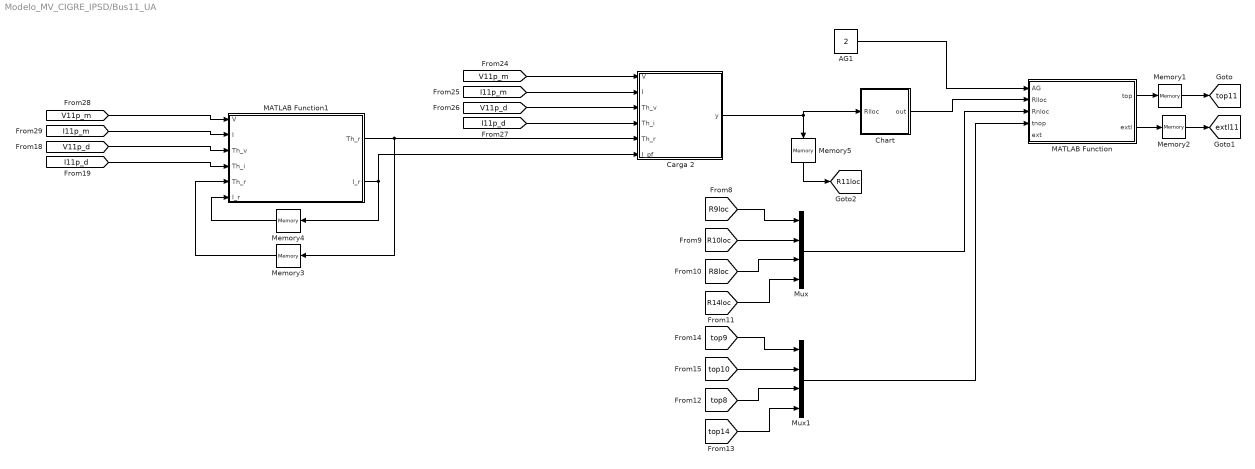
== system Modelo_MV_CIGRE_IPSD/Bus11_UA ==
  AG1 : Constant  Value=2
  Carga 2 : MATLAB Function  TreatAsAtomicUnit=on
  Chart : Stateflow chart  BlockKeywords=__PRM__SERIALIZED__DATA__:Stateflow Chart,Stateflow Diagram  TreatAsAtomicUnit=on
  MATLAB Function : MATLAB Function  TreatAsAtomicUnit=on
  MATLAB Function1 : MATLAB Function  TreatAsAtomicUnit=on
  Memory{1..5} (5 alike) : Memory
  Mux : Mux
  Mux1 : Mux
  tag scope: R11loc=global, extl11=global, top11=global
  wires:
  AG1/1 -> MATLAB Function/1(AG)
  MATLAB Function/1(top) -> Memory1/1
  MATLAB Function/2(extl) -> Memory2/1
  MATLAB Function1/2(I_r) -> Carga 2/6(I_pf), Memory4/1
  Memory3/1 -> MATLAB Function1/5("Th_r ")
  [V11p_d] -> MATLAB Function1/3(Th_v)
  [I11p_d] -> Carga 2/4(Th_i)
  Memory4/1 -> MATLAB Function1/6("I_r ")
  [I11p_d] -> MATLAB Function1/4(Th_i)
  [V11p_d] -> Carga 2/3(Th_v)
  MATLAB Function1/1(Th_r) -> Carga 2/5(Th_r), Memory3/1
  [I11p_m] -> MATLAB Function1/2(I)
  [V11p_m] -> Carga 2/1(V)
  [I11p_m] -> Carga 2/2(I)
  [V11p_m] -> MATLAB Function1/1(V)
  Carga 2/1(y) -> Chart/1(Rlloc), Memory5/1
  [top9] -> Mux1/1
  [top10] -> Mux1/2
  [top8] -> Mux1/3
  Mux/1 -> MATLAB Function/3(Rnloc)
  [top14] -> Mux1/4
  [R10loc] -> Mux/2
  [R8loc] -> Mux/3
  [R9loc] -> Mux/1
  Mux1/1 -> MATLAB Function/4(tnop)
  [R14loc] -> Mux/4
  Memory1/1 -> [top11]
  Memory2/1 -> [extl11]
  Memory5/1 -> [R11loc]
  Chart/1(out) -> MATLAB Function/2(Rlloc)

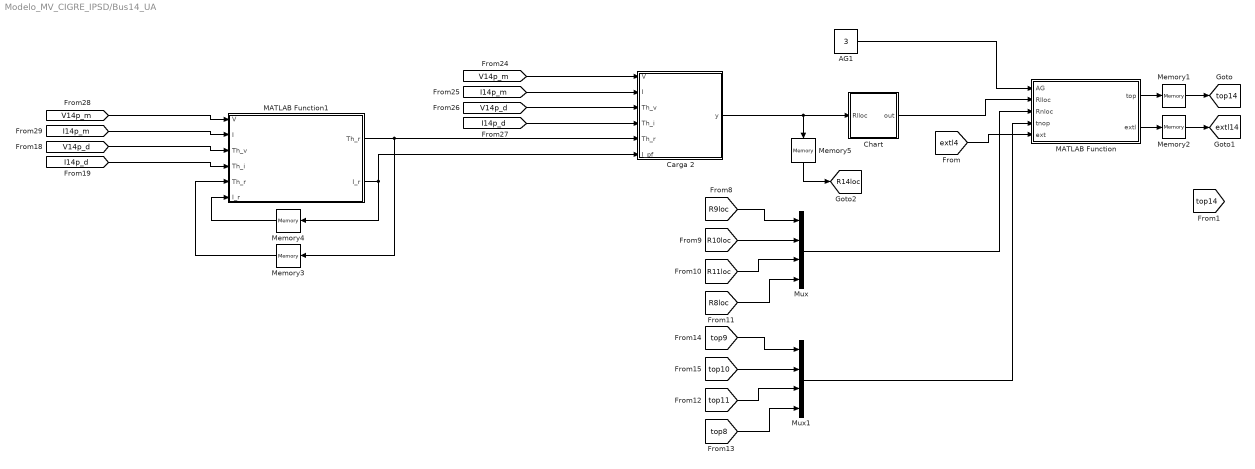
== system Modelo_MV_CIGRE_IPSD/Bus14_UA ==
  AG1 : Constant  Value=3
  Carga 2 : MATLAB Function  TreatAsAtomicUnit=on
  Chart : Stateflow chart  BlockKeywords=__PRM__SERIALIZED__DATA__:Stateflow Chart,Stateflow Diagram  TreatAsAtomicUnit=on
  MATLAB Function : MATLAB Function  TreatAsAtomicUnit=on
  MATLAB Function1 : MATLAB Function  TreatAsAtomicUnit=on
  Memory{1..5} (5 alike) : Memory
  Mux : Mux
  Mux1 : Mux
  tag scope: R14loc=global, extl14=global, top14=global
  wires:
  AG1/1 -> MATLAB Function/1(AG)
  MATLAB Function/1(top) -> Memory1/1
  MATLAB Function/2(extl) -> Memory2/1
  MATLAB Function1/2(I_r) -> Carga 2/6(I_pf), Memory4/1
  Memory3/1 -> MATLAB Function1/5("Th_r ")
  [V14p_d] -> MATLAB Function1/3(Th_v)
  [I14p_d] -> Carga 2/4(Th_i)
  Memory4/1 -> MATLAB Function1/6("I_r ")
  [I14p_d] -> MATLAB Function1/4(Th_i)
  [V14p_d] -> Carga 2/3(Th_v)
  MATLAB Function1/1(Th_r) -> Carga 2/5(Th_r), Memory3/1
  [I14p_m] -> MATLAB Function1/2(I)
  [V14p_m] -> Carga 2/1(V)
  [I14p_m] -> Carga 2/2(I)
  [V14p_m] -> MATLAB Function1/1(V)
  Carga 2/1(y) -> Chart/1(Rlloc), Memory5/1
  [top9] -> Mux1/1
  [top10] -> Mux1/2
  [top11] -> Mux1/3
  Mux/1 -> MATLAB Function/3(Rnloc)
  [top8] -> Mux1/4
  [R10loc] -> Mux/2
  [R11loc] -> Mux/3
  [R9loc] -> Mux/1
  Mux1/1 -> MATLAB Function/4(tnop)
  [R8loc] -> Mux/4
  [extl4] -> MATLAB Function/5(ext)
  Memory1/1 -> [top14]
  Memory2/1 -> [extl14]
  Memory5/1 -> [R14loc]
  Chart/1(out) -> MATLAB Function/2(Rlloc)

== system Modelo_MV_CIGRE_IPSD/Bus15_UA ==
  AG1 : Constant  Value=2
  Carga 2 : MATLAB Function  TreatAsAtomicUnit=on
  Chart : Stateflow chart  BlockKeywords=__PRM__SERIALIZED__DATA__:Stateflow Chart,Stateflow Diagram  TreatAsAtomicUnit=on
  MATLAB Function : MATLAB Function  TreatAsAtomicUnit=on
  MATLAB Function1 : MATLAB Function  TreatAsAtomicUnit=on
  Memory{1..5} (5 alike) : Memory
  Mux : Mux  Inputs=3
  Mux1 : Mux  Inputs=3
  tag scope: R15loc=global, extl15=global, top15=global
  wires:
  AG1/1 -> MATLAB Function/1(AG)
  MATLAB Function/1(top) -> Memory1/1
  MATLAB Function/2(extl) -> Memory2/1
  [I15p_m] -> Carga 2/2(I)
  [V15p_m] -> Carga 2/1(V)
  MATLAB Function1/1(Th_r) -> Carga 2/5(Th_r), Memory3/1
  [V15p_d] -> Carga 2/3(Th_v)
  [I15p_d] -> Carga 2/4(Th_i)
  Memory4/1 -> MATLAB Function1/6("I_r ")
  MATLAB Function1/2(I_r) -> Carga 2/6(I_pf), Memory4/1
  Carga 2/1(y) -> Chart/1(Rlloc), Memory5/1
  Memory3/1 -> MATLAB Function1/5("Th_r ")
  [V15p_m] -> MATLAB Function1/1(V)
  [I15p_m] -> MATLAB Function1/2(I)
  [V15p_d] -> MATLAB Function1/3(Th_v)
  [I15p_d] -> MATLAB Function1/4(Th_i)
  [R4loc] -> Mux/3
  Mux1/1 -> MATLAB Function/4(tnop)
  [R3loc] -> Mux/2
  [top2] -> Mux1/1
  [R2loc] -> Mux/1
  Mux/1 -> MATLAB Function/3(Rnloc)
  [top4] -> Mux1/3
  [top3] -> Mux1/2
  Memory1/1 -> [top15]
  Memory2/1 -> [extl15]
  Memory5/1 -> [R15loc]
  Chart/1(out) -> MATLAB Function/2(Rlloc)

== system Modelo_MV_CIGRE_IPSD/Bus2_UA ==
  AG1 : Constant  Value=2
  Carga 2 : MATLAB Function  TreatAsAtomicUnit=on
  Chart : Stateflow chart  BlockKeywords=__PRM__SERIALIZED__DATA__:Stateflow Chart,Stateflow Diagram  TreatAsAtomicUnit=on
  MATLAB Function : MATLAB Function  TreatAsAtomicUnit=on
  MATLAB Function1 : MATLAB Function  TreatAsAtomicUnit=on
  Memory{1..5} (5 alike) : Memory
  Mux : Mux  Inputs=3
  Mux1 : Mux  Inputs=3
  tag scope: R2loc=global, extl2=global, top2=global
  wires:
  AG1/1 -> MATLAB Function/1(AG)
  MATLAB Function/1(top) -> Memory2/1
  MATLAB Function/2(extl) -> Memory5/1
  [I2p_m] -> Carga 2/2(I)
  [V2p_m] -> Carga 2/1(V)
  MATLAB Function1/1(Th_r) -> Carga 2/5(Th_r), Memory3/1
  [V2p_d] -> Carga 2/3(Th_v)
  [I2p_d] -> Carga 2/4(Th_i)
  Memory4/1 -> MATLAB Function1/6("I_r ")
  MATLAB Function1/2(I_r) -> Carga 2/6(I_pf), Memory4/1
  Carga 2/1(y) -> Chart/1(Rlloc), Memory1/1
  Memory3/1 -> MATLAB Function1/5("Th_r ")
  [V2p_m] -> MATLAB Function1/1(V)
  [I2p_m] -> MATLAB Function1/2(I)
  [V2p_d] -> MATLAB Function1/3(Th_v)
  [I2p_d] -> MATLAB Function1/4(Th_i)
  [R15loc] -> Mux/3
  Mux1/1 -> MATLAB Function/4(tnop)
  [R3loc] -> Mux/2
  [top4] -> Mux1/1
  [R4loc] -> Mux/1
  Mux/1 -> MATLAB Function/3(Rnloc)
  [top15] -> Mux1/3
  [top3] -> Mux1/2
  Memory1/1 -> [R2loc]
  Memory2/1 -> [top2]
  Memory5/1 -> [extl2]
  Chart/1(out) -> MATLAB Function/2(Rlloc)

== system Modelo_MV_CIGRE_IPSD/Bus3_UA ==
  AG1 : Constant  Value=2
  Carga 2 : MATLAB Function  TreatAsAtomicUnit=on
  Chart : Stateflow chart  BlockKeywords=__PRM__SERIALIZED__DATA__:Stateflow Chart,Stateflow Diagram  TreatAsAtomicUnit=on
  MATLAB Function : MATLAB Function  TreatAsAtomicUnit=on
  MATLAB Function1 : MATLAB Function  TreatAsAtomicUnit=on
  Memory{1..5} (5 alike) : Memory
  Mux : Mux  Inputs=3
  Mux1 : Mux  Inputs=3
  tag scope: R3loc=global, extl3=global, top3=global
  wires:
  AG1/1 -> MATLAB Function/1(AG)
  MATLAB Function/1(top) -> Memory2/1
  MATLAB Function/2(extl) -> Memory5/1
  [I3p_m] -> Carga 2/2(I)
  [V3p_m] -> Carga 2/1(V)
  MATLAB Function1/1(Th_r) -> Carga 2/5(Th_r), Memory3/1
  [V3p_d] -> Carga 2/3(Th_v)
  [I3p_d] -> Carga 2/4(Th_i)
  Memory4/1 -> MATLAB Function1/6("I_r ")
  MATLAB Function1/2(I_r) -> Carga 2/6(I_pf), Memory4/1
  Carga 2/1(y) -> Chart/1(Rlloc), Memory1/1
  Memory3/1 -> MATLAB Function1/5("Th_r ")
  [V3p_m] -> MATLAB Function1/1(V)
  [I3p_m] -> MATLAB Function1/2(I)
  [V3p_d] -> MATLAB Function1/3(Th_v)
  [I3p_d] -> MATLAB Function1/4(Th_i)
  [R15loc] -> Mux/3
  Mux1/1 -> MATLAB Function/4(tnop)
  [R4loc] -> Mux/2
  [top2] -> Mux1/1
  [R2loc] -> Mux/1
  Mux/1 -> MATLAB Function/3(Rnloc)
  [top15] -> Mux1/3
  [top4] -> Mux1/2
  Memory1/1 -> [R3loc]
  Memory2/1 -> [top3]
  Memory5/1 -> [extl3]
  Chart/1(out) -> MATLAB Function/2(Rlloc)

== system Modelo_MV_CIGRE_IPSD/Bus4_UA ==
  AG1 : Constant  Value=3
  Carga 2 : MATLAB Function  TreatAsAtomicUnit=on
  Chart : Stateflow chart  BlockKeywords=__PRM__SERIALIZED__DATA__:Stateflow Chart,Stateflow Diagram  TreatAsAtomicUnit=on
  MATLAB Function : MATLAB Function  TreatAsAtomicUnit=on
  MATLAB Function1 : MATLAB Function  TreatAsAtomicUnit=on
  Memory{1..5} (5 alike) : Memory
  Mux : Mux  Inputs=3
  Mux1 : Mux  Inputs=3
  tag scope: R4loc=global, extl4=global, top4=global
  wires:
  AG1/1 -> MATLAB Function/1(AG)
  MATLAB Function/1(top) -> Memory2/1
  MATLAB Function/2(extl) -> Memory5/1
  [I4p_m] -> Carga 2/2(I)
  [V4p_m] -> Carga 2/1(V)
  MATLAB Function1/1(Th_r) -> Carga 2/5(Th_r), Memory3/1
  [V4p_d] -> Carga 2/3(Th_v)
  [I4p_d] -> Carga 2/4(Th_i)
  Memory4/1 -> MATLAB Function1/6("I_r ")
  MATLAB Function1/2(I_r) -> Carga 2/6(I_pf), Memory4/1
  Carga 2/1(y) -> Chart/1(Rlloc), Memory1/1
  Memory3/1 -> MATLAB Function1/5("Th_r ")
  [V4p_m] -> MATLAB Function1/1(V)
  [I4p_m] -> MATLAB Function1/2(I)
  [V4p_d] -> MATLAB Function1/3(Th_v)
  [I4p_d] -> MATLAB Function1/4(Th_i)
  [top2] -> Mux1/1
  [top3] -> Mux1/2
  [top15] -> Mux1/3
  Mux/1 -> MATLAB Function/3(Rnloc)
  [R3loc] -> Mux/2
  [R15loc] -> Mux/3
  [R2loc] -> Mux/1
  Mux1/1 -> MATLAB Function/4(tnop)
  [extl14] -> MATLAB Function/5(ext)
  Memory1/1 -> [R4loc]
  Memory2/1 -> [top4]
  Memory5/1 -> [extl4]
  Chart/1(out) -> MATLAB Function/2(Rlloc)

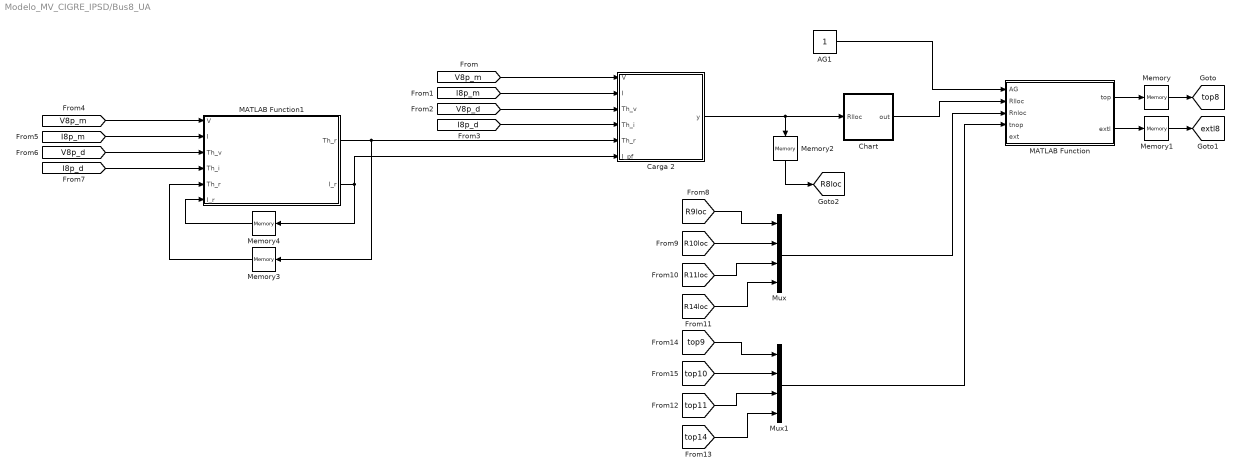
== system Modelo_MV_CIGRE_IPSD/Bus8_UA ==
  AG1 : Constant
  Carga 2 : MATLAB Function  TreatAsAtomicUnit=on
  Chart : Stateflow chart  BlockKeywords=__PRM__SERIALIZED__DATA__:Stateflow Chart,Stateflow Diagram  TreatAsAtomicUnit=on
  MATLAB Function : MATLAB Function  TreatAsAtomicUnit=on
  MATLAB Function1 : MATLAB Function  TreatAsAtomicUnit=on
  Memory{,1..4} (5 alike) : Memory
  Mux : Mux
  Mux1 : Mux
  tag scope: R8loc=global, extl8=global, top8=global
  wires:
  AG1/1 -> MATLAB Function/1(AG)
  MATLAB Function/1(top) -> Memory/1
  MATLAB Function/2(extl) -> Memory1/1
  [I8p_m] -> Carga 2/2(I)
  [V8p_m] -> Carga 2/1(V)
  MATLAB Function1/1(Th_r) -> Memory3/1, Carga 2/5(Th_r)
  [V8p_d] -> Carga 2/3(Th_v)
  [I8p_d] -> Carga 2/4(Th_i)
  Memory4/1 -> MATLAB Function1/6("I_r ")
  MATLAB Function1/2(I_r) -> Memory4/1, Carga 2/6(I_pf)
  Carga 2/1(y) -> Chart/1(Rlloc), Memory2/1
  Memory3/1 -> MATLAB Function1/5("Th_r ")
  [V8p_m] -> MATLAB Function1/1(V)
  [I8p_m] -> MATLAB Function1/2(I)
  [V8p_d] -> MATLAB Function1/3(Th_v)
  [I8p_d] -> MATLAB Function1/4(Th_i)
  [R9loc] -> Mux/1
  [R10loc] -> Mux/2
  [R11loc] -> Mux/3
  [R14loc] -> Mux/4
  Mux/1 -> MATLAB Function/3(Rnloc)
  Mux1/1 -> MATLAB Function/4(tnop)
  [top10] -> Mux1/2
  [top11] -> Mux1/3
  [top9] -> Mux1/1
  [top14] -> Mux1/4
  Memory/1 -> [top8]
  Memory1/1 -> [extl8]
  Memory2/1 -> [R8loc]
  Chart/1(out) -> MATLAB Function/2(Rlloc)

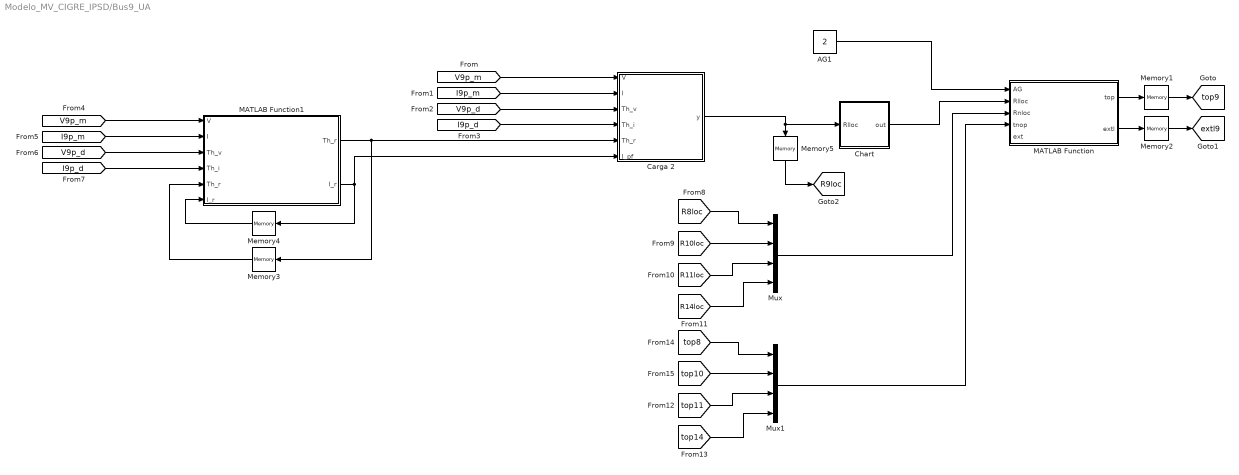
== system Modelo_MV_CIGRE_IPSD/Bus9_UA ==
  AG1 : Constant  Value=2
  Carga 2 : MATLAB Function  TreatAsAtomicUnit=on
  Chart : Stateflow chart  BlockKeywords=__PRM__SERIALIZED__DATA__:Stateflow Chart,Stateflow Diagram  TreatAsAtomicUnit=on
  MATLAB Function : MATLAB Function  TreatAsAtomicUnit=on
  MATLAB Function1 : MATLAB Function  TreatAsAtomicUnit=on
  Memory{1..5} (5 alike) : Memory
  Mux : Mux
  Mux1 : Mux
  tag scope: R9loc=global, extl9=global, top9=global
  wires:
  AG1/1 -> MATLAB Function/1(AG)
  MATLAB Function/1(top) -> Memory1/1
  MATLAB Function/2(extl) -> Memory2/1
  [I9p_m] -> Carga 2/2(I)
  [V9p_m] -> Carga 2/1(V)
  MATLAB Function1/1(Th_r) -> Carga 2/5(Th_r), Memory3/1
  [V9p_d] -> Carga 2/3(Th_v)
  [I9p_d] -> Carga 2/4(Th_i)
  Memory4/1 -> MATLAB Function1/6("I_r ")
  MATLAB Function1/2(I_r) -> Carga 2/6(I_pf), Memory4/1
  Carga 2/1(y) -> Chart/1(Rlloc), Memory5/1
  Memory3/1 -> MATLAB Function1/5("Th_r ")
  [V9p_m] -> MATLAB Function1/1(V)
  [I9p_m] -> MATLAB Function1/2(I)
  [V9p_d] -> MATLAB Function1/3(Th_v)
  [I9p_d] -> MATLAB Function1/4(Th_i)
  [top8] -> Mux1/1
  [top10] -> Mux1/2
  [top11] -> Mux1/3
  Mux/1 -> MATLAB Function/3(Rnloc)
  [top14] -> Mux1/4
  [R10loc] -> Mux/2
  [R11loc] -> Mux/3
  [R8loc] -> Mux/1
  Mux1/1 -> MATLAB Function/4(tnop)
  [R14loc] -> Mux/4
  Memory1/1 -> [top9]
  Memory2/1 -> [extl9]
  Memory5/1 -> [R9loc]
  Chart/1(out) -> MATLAB Function/2(Rlloc)

== system Modelo_MV_CIGRE_IPSD/DER ==
  Control IBRs : Subsystem
  Controlled Voltage Source : powerlib/Electrical Sources/Controlled Voltage Source  Initialize=on  Source_Type=AC  Amplitude=400*sqrt(2/3)  Phase=0  Frequency=60  Measurements=None
      settings: SourceProductName=Simscape Electrical
  Controlled Voltage Source2 : powerlib/Electrical Sources/Controlled Voltage Source  Initialize=on  Source_Type=AC  Amplitude=400*sqrt(2/3)  Phase=120  Frequency=60  Measurements=None
      settings: SourceProductName=Simscape Electrical
  Controlled Voltage Source3 : powerlib/Electrical Sources/Controlled Voltage Source  Initialize=on  Source_Type=AC  Amplitude=400*sqrt(2/3)  Phase=-120  Frequency=60  Measurements=None
      settings: SourceProductName=Simscape Electrical
  Ground : powerlib/Elements/Ground  LConnTagsString=a
      settings: SourceProductName=Simscape Electrical
  "Power (3ph, Instantaneous)" : powerlib_meascontrol/Measurements/Power (3ph, Instantaneous)
      settings: SourceProductName=Simscape Electrical
  Scope : Scope
  Scope1 : Scope  NumInputPorts=2
  Scope4 : Scope  NumInputPorts=3
  Scope5 : Scope
  Scope6 : Scope
  Three-Phase Series RLC Branch1 : powerlib/Elements/Three-Phase Series RLC Branch  LConnTagsString=A|B|C  RConnTagsString=A|B|C  BranchType=RL  Resistance=0.57  Inductance=1.5e-3  Capacitance=1e-6  Measurements=None
      settings: SourceProductName=Simscape Electrical
  Three-Phase Series RLC Branch2 : powerlib/Elements/Three-Phase Series RLC Branch  LConnTagsString=A|B|C  RConnTagsString=A|B|C  BranchType=C  Resistance=0.01  Inductance=1e-3  Capacitance=3e-6  Measurements=None
      settings: SourceProductName=Simscape Electrical
  Three-Phase V-I Measurement : powerlib/Measurements/Three-Phase V-I Measurement  VoltageMeasurement=phase-to-ground  SetLabelV=on  LabelV=Vabc_DER1  Vpu=on  VpuLL=off  CurrentMeasurement=yes  SetLabelI=on  LabelI=Iabc_DER1  Ipu=on  Pbase=100e3  Vbase=400  OutputType=Complex  PhasorSimulation=off  PSBequivalent=0
      settings: SourceProductName=Simscape Electrical
  Three-Phase Source : powerlib/Electrical Sources/Three-Phase Source  InternalConnection=Y  VoltagePhases=off  Voltage=400  PhaseAngle=0  Voltage_phases=[25e3 25e3 25e3]/sqrt(3)  PhaseAngles_phases=[0 -120 +120]  Frequency=60  NonIdealSource=on  SpecifyImpedance=on  Resistance=0.8929  Inductance=16.58e-3  ShortCircuitLevel=10e3  BaseVoltage=400  XRratio=7  BusType=swing  Pref=10e3  Qref=0  Prefabc=[10e3, 10e3, 10e3]  Qrefabc=[0, 0, 0]  Qmin=-inf  Qmax=inf
      settings: SourceProductName=Simscape Electrical
  Three-Phase Transformer Inductance Matrix Type (Two Windings) : powerlib/Elements/Three-Phase Transformer Inductance Matrix Type (Two Windings)  CoreType=Three single-phase cores  Winding1Connection=Yg  Winding2Connection=Delta (D1)  AutoTransformer=off  Measurements=None  NominalPower=[300e3, 60]  VLLnom=[20e3, 400]  WindingResistances=[0.01, 0.01]  NoLoadIexcPos=2  NoLoadPlossPos=1000  ShortCircuitReactancePos=0.06  ShortCircuitReactancePosAuto=0.06  NoLoadIexcZero=100  NoLoadPlossZero=1500  ShortCircuitReactanceZero=0.03  ShortCircuitReactanceZeroAuto=0.03
      settings: SourceProductName=Simscape Electrical  SourceProductBaseCode=PS
  A : PMIOPort  Side=Left
  B : PMIOPort  Port=2  Side=Left
  C : PMIOPort  Port=3  Side=Left
  wires:
  Control IBRs/2(Vb) -> Scope4/2, Controlled Voltage Source2/1
  [Vabc_DER1] -> "Power (3ph, Instantaneous)"/1, Scope/1, Scope1/2, Control IBRs/1(Vmeas)
  Control IBRs/3(Vc) -> Scope4/3, Controlled Voltage Source3/1
  "Power (3ph, Instantaneous)"/1 -> Scope5/1
  Control IBRs/1(Va) -> Scope4/1, Controlled Voltage Source/1
  "Power (3ph, Instantaneous)"/2 -> Scope6/1
  [Iabc_DER1] -> Scope1/1, "Power (3ph, Instantaneous)"/2, Control IBRs/2(Imeas)
  connections:
  Ground/LConn1 -- Three-Phase Series RLC Branch2/RConn1 -- Three-Phase Series RLC Branch2/RConn3 -- Controlled Voltage Source/LConn1 -- Controlled Voltage Source2/LConn1 -- Controlled Voltage Source3/LConn1 -- Three-Phase Series RLC Branch2/RConn2
  C/RConn1 -- Three-Phase Transformer Inductance Matrix Type (Two Windings)/LConn3
  Three-Phase Series RLC Branch1/RConn1 -- Controlled Voltage Source/RConn1
  Three-Phase Transformer Inductance Matrix Type (Two Windings)/RConn3 -- Three-Phase Source/RConn3 -- Three-Phase V-I Measurement/RConn3
  Three-Phase Transformer Inductance Matrix Type (Two Windings)/LConn2 -- B/RConn1
  Three-Phase Series RLC Branch1/LConn3 -- Three-Phase V-I Measurement/LConn3 -- Three-Phase Series RLC Branch2/LConn3
  Three-Phase Series RLC Branch1/RConn2 -- Controlled Voltage Source2/RConn1
  Three-Phase Series RLC Branch1/LConn1 -- Three-Phase V-I Measurement/LConn1 -- Three-Phase Series RLC Branch2/LConn1
  Three-Phase V-I Measurement/RConn1 -- Three-Phase Source/RConn1 -- Three-Phase Transformer Inductance Matrix Type (Two Windings)/RConn1
  Three-Phase V-I Measurement/RConn2 -- Three-Phase Source/RConn2 -- Three-Phase Transformer Inductance Matrix Type (Two Windings)/RConn2
  Three-Phase Series RLC Branch1/RConn3 -- Controlled Voltage Source3/RConn1
  Three-Phase Series RLC Branch1/LConn2 -- Three-Phase Series RLC Branch2/LConn2 -- Three-Phase V-I Measurement/LConn2
  A/RConn1 -- Three-Phase Transformer Inductance Matrix Type (Two Windings)/LConn1
